simulink model "non_linear_simulation_v2"  (R2020a)
settings: Solver=ode4  StartTime=0.0  StopTime=inf  FixedStep=0.01  RelTol=1e-3
InitFcn:
  | run('initialize_system.m')
values from neighbouring files (symbols this model uses):
  Ac = [d_f1_dth,d_f1_dyw,d_f1_dw_th,d_f1_dw_yw ... (first row only)    [linearize_heli.m]
  Bc = [d_f1_Vmp,d_f1_Vmy ... (first row only)    [linearize_heli.m]
  Cc = [1,0,0,0;0,1,0,0]    [linearize_heli.m]
  Q = diag([5e1,7e1,8e1,6e1])    [initialize_system.m]
  R = diag([0.1,0.1])    [initialize_system.m]
  th_op = -30*pi/180    (= -0.523598775598)    [initialize_system.m]
  Vmp_op = (Kyy*m_heli*g*cos(th_op)*l_cm) / (Kyy*Kpp - Kyp*Kpy)    [initialize_system.m]
  Vmy_op = (Kyp*Vmp_op) / (Kyy)    [initialize_system.m]
  w_th_op = 0    [initialize_system.m]
  w_yw_op = 0    [initialize_system.m]
  yw_op = pi/2    (= 1.57079632679)    [initialize_system.m]
undefined symbols (not defined in the file or in its folder): L, P0
libraries: realtime_pacer_lib x1, dspsigops x1
(part 2 of 2)

== matlab function non_linear_simulation_v2/nonlinear_model ==
  data: Vmp input; d_th_dt output; Vmy input; th input; yw input; w_th input; w_yw input; d_yw_dt output; d_w_th_dt output; d_w_yw_dt output
% Simulink nonlinear model of USN helicopter
% Author: Eirik Engen
% Date: 2020-09-02

function [d_th_dt, d_yw_dt, d_w_th_dt, d_w_yw_dt] = non_linear_model(Vmp, Vmy, th, yw, w_th, w_yw)          %#ok<INUSL>
% function inputs
% Vmp : Model input - Voltage input to Pitch motor/rotor [V]
% Vmy : Model input - Voltage input to Yaw motor/rotor [V]
% th  : Model state - Pitch angle, theta [radians]
% yw  : Model state - Yaw angle, psi [radians]
% w_th: Model state - Pitch angular velocity, omega_theta [radians / s]
% w_yw: Model state - Yaw angular velocity, omega_psi [radians / s]

% System parameters
l_cm   = 0.015;   % [m] - Distance between the pivot point and the center of mass of the helicopter.
m_heli = 0.479;   % [kg] - Total moving mass of the helicopter
J_eq_p = 0.0172;  % [kg-m^2] - Moment of inertia about pitch axis
J_eq_y = 0.0210;  % [kg-m^2] - Moment of inertia about yaw axis
g      = 9.81;    % [m/s^2] - Acceleration due to gravity on planet earth

Kpp    = 0.0556;  % [Nm/V] - Torque constant on pitch axis from pitch motor
Kyy    = 0.21084; % [Nm/V] - Torque constant on yaw axis from yaw motor
Kpy    = 0.005;   % [Nm/V] - Torque constant on pitch axis from yaw motor
Kyp    = 0.15;    % [Nm/V] - Torque constant on yaw axis from pitch motor
Bp     = 0.01;    % [N/V]  - Damping friction factor about pitch axis
By     = 0.08;    % [N/V]  - Damping friction factor about yaw axis

% Differential equations
d_th_dt = w_th;
d_yw_dt = w_yw;
d_w_th_dt = (Kpp*Vmp - ...
    Kpy*Vmy - ...
    Bp*w_th - ...
    m_heli*l_cm^2*w_yw^2*sin(th)*cos(th) - ...
    m_heli*g*l_cm*cos(th)) / ...
    (J_eq_p+m_heli*l_cm^2);
d_w_yw_dt = (Kyp*Vmp - ...
    Kyy*Vmy - ...
    By*w_yw + ...
    2*m_heli*l_cm^2*w_th*w_yw*sin(th)*cos(th)) / ...
    (J_eq_y+m_heli*l_cm^2*cos(th)^2);
